simulink model "ventilator_LungBreathingCircuit2"  (R2020a)
settings: Solver=VariableStepAuto  StartTime=0.0  StopTime=30  RelTol=1e-9  AbsTol=1e-8
PostLoadFcn:
  | hws = get_param(bdroot, 'modelworkspace');
  | hws.assignin('T_room', 20); % degC
  | hws.assignin('RH_room', 0.1); % degC
  | hws.assignin('T_humidifier', 40); % degC
  | hws.assignin('T_body', 37); % degC
  | 
  | hws.assignin('L_tube', 1); % m
  | hws.assignin('D_tube', 0.01); % m
  | hws.assignin('L_trachea', 0.15); % m
  | hws.assignin('D_trachea', 0.015); % m
  | 
  | % Conversion factors
  | hws.assignin('cmH2O_to_Pa', 98.0665);
  | hws.assignin('L_to_m3', 1e-3);
  | 
  | % L Functional Residual Capacity https://www.ncbi.nlm.nih.gov/books/NBK500007/
  | hws.assignin('FRC', 2);
  | hws.assignin('C_respiratory', 50); % mL/cmH2O
  | hws.assignin('R_respiratory', 5); % cmH2O/(L/s)
  | hws.assignin('P_muscle', 0); % cmH2O
  | %E_respiratory = 20; % cmH2O/L    C_respiratory = 1/E_respiratory * 1000;
  | % http://www.ubccriticalcaremedicine.ca/rotating/material/Lecture_1%20for%20Residents.pdf
  | 
  | clear hws;
model workspace (MAT data in the model file):
  C_respiratory = 50
  D_trachea = 0.015
  D_tube = 0.01
  FRC = 2
  L_to_m3 = 0.001
  L_trachea = 0.15
  L_tube = 1
  P_muscle = 0
  RH_room = 0.1
  R_respiratory = 5
  T_body = 37
  T_humidifier = 40
  T_room = 20
  cmH2O_to_Pa = 98.0665
libraries: fl_lib x56, nesl_utility x8, simulink x1
(part 2 of 2)

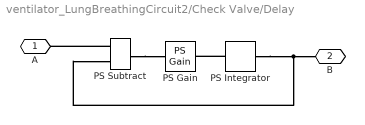
== system ventilator_LungBreathingCircuit2/Check Valve/Delay ==
  PS Gain : fl_lib/Physical Signals/Functions/PS Gain  gain=1/tau 1/s
  PS Integrator : fl_lib/Physical Signals/Linear Operators/PS Integrator  x0=x0 m^2
      settings: SourceProductBaseCode=SS
  PS Subtract : fl_lib/Physical Signals/Functions/PS Subtract
  A : PMIOPort  Side=Left
  B : PMIOPort  Port=2  Side=Right
  connections:
  PS Integrator/RConn1 -- PS Subtract/LConn2 -- B/RConn1
  PS Subtract/RConn1 -- PS Gain/LConn1
  PS Subtract/LConn1 -- A/RConn1
  PS Integrator/LConn1 -- PS Gain/RConn1

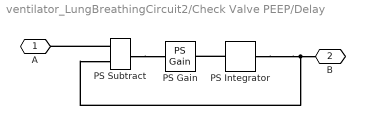
== system ventilator_LungBreathingCircuit2/Check Valve PEEP/Delay ==
  PS Gain : fl_lib/Physical Signals/Functions/PS Gain  gain=1/tau 1/s
  PS Integrator : fl_lib/Physical Signals/Linear Operators/PS Integrator  x0=x0 m^2
      settings: SourceProductBaseCode=SS
  PS Subtract : fl_lib/Physical Signals/Functions/PS Subtract
  A : PMIOPort  Side=Left
  B : PMIOPort  Port=2  Side=Right
  connections:
  PS Integrator/LConn1 -- PS Gain/RConn1
  PS Subtract/LConn1 -- A/RConn1
  PS Subtract/RConn1 -- PS Gain/LConn1
  B/RConn1 -- PS Subtract/LConn2 -- PS Integrator/RConn1

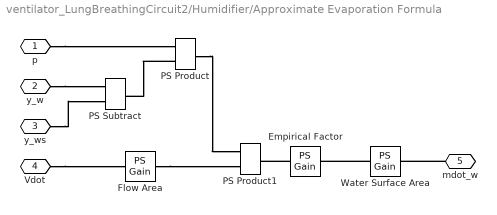
== system ventilator_LungBreathingCircuit2/Humidifier/Approximate Evaporation Formula ==
  Empirical Factor : fl_lib/Physical Signals/Functions/PS Gain  gain=5e-8 kg/J
  Flow Area : fl_lib/Physical Signals/Functions/PS Gain  gain=1 / (pi*D_tube^2/4) 1/m^2
  PS Product : fl_lib/Physical Signals/Functions/PS Product
  PS Product1 : fl_lib/Physical Signals/Functions/PS Product
  PS Subtract : fl_lib/Physical Signals/Functions/PS Subtract
  Water Surface Area : fl_lib/Physical Signals/Functions/PS Gain  gain=A_humidifier m^2
  p : PMIOPort  Side=Left
  y_w : PMIOPort  Port=2  Side=Left
  y_ws : PMIOPort  Port=3  Side=Left
  Vdot : PMIOPort  Port=4  Side=Left
  mdot_w : PMIOPort  Port=5  Side=Right
  connections:
  y_w/RConn1 -- PS Subtract/LConn2
  y_ws/RConn1 -- PS Subtract/LConn1
  p/RConn1 -- PS Product/LConn1
  PS Product/LConn2 -- PS Subtract/RConn1
  PS Product/RConn1 -- PS Product1/LConn1
  Flow Area/RConn1 -- PS Product1/LConn2
  Empirical Factor/LConn1 -- PS Product1/RConn1
  Water Surface Area/LConn1 -- Empirical Factor/RConn1
  mdot_w/RConn1 -- Water Surface Area/RConn1
  Vdot/RConn1 -- Flow Area/LConn1

== matlab function ventilator_LungBreathingCircuit2/Flow Profile/MATLAB Function ==
  data: t input; inhale output; exhale output; respiratory_rate parameter; IE parameter; input_pressure parameter; D_tube parameter; TAIP parameter
function [inhale, exhale] = fcn(t,respiratory_rate, IE, input_pressure,  D_tube, TAIP)

% Define timing constants
T_period        = 60 / respiratory_rate;
T_inspiration   = 1 / (IE+1) * T_period;
T_inhale_hold   = 0.1;
%T_exhale       = T_period - T_inspiration;

cycle_timer  = rem(t,T_period);
duration = (T_inspiration - T_inhale_hold);
TAIP = TAIP/100;
input_pressure = input_pressure*98.0665;

if TAIP == 0 % Ideal TAIP
    if cycle_timer <= duration
        inhale = 1;
        exhale = 0;
    elseif cycle_timer < T_inspiration
        inhale = 0;
        exhale = 0;
    else
        inhale = 0;
        exhale = 1;
    end
elseif TAIP > 0 % TAIP
    if cycle_timer <= duration
        inhale_max = 2;    % Height for a triangle is twice of a square with similar base and same area
        if cycle_timer <= duration
            slope =  inhale_max / (TAIP/2);   % accelerating
            t     =  cycle_timer - 0;
        else
            slope = 0;   % deccelerating
            t     = cycle_timer - duration;
        end
        if t > 0.9
            a= 1;
        end
        inhale = slope * t;
        exhale = 0;
    elseif cycle_timer < T_inspiration
        inhale = 0;
        exhale = 0;
    else
        inhale = 0;
        exhale = 1;
    end
else
    % Default values for Simulink
    inhale = 0;
    exhale = 0;
end
MaxValveArea = pi*D_tube^2/4;

inhale = inhale*input_pressure;
exhale = exhale * MaxValveArea * input_pressure;
